simulink model "P_vertical"  (R2017b)
settings: Solver=VariableStepAuto  StartTime=0.0  StopTime=10.0  RelTol=1e-3
libraries: simulink x1
settings Model: Creator=Rita Monteiro  LastModifiedBy=Rita Monteiro

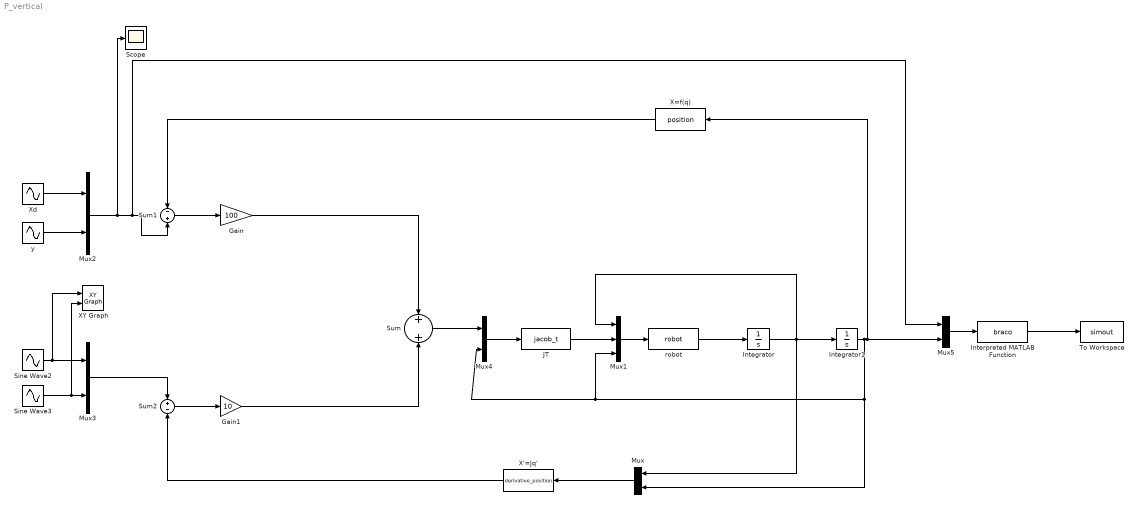
== system P_vertical ==
  Gain : Gain  Gain=100
  Gain1 : Gain  Gain=10
  Integrator : Integrator  InitialCondition=[0;0]
  Integrator1 : Integrator  InitialCondition=[pi/2;-pi/4]
  Interpreted MATLAB Function : MATLABFcn  MATLABFcn=braco  OutputDimensions=1
  JT : MATLABFcn  MATLABFcn=jacob_t  OutputDimensions=2
  Mux{,2..5} (5 alike) : Mux  Inputs=2
  Mux1 : Mux  Inputs=3
  Scope : Scope
  Sine Wave2 : Sin  Amplitude=0  Frequency=2*pi*0.25  Phase=pi  SampleTime=0
  Sine Wave3 : Sin  Amplitude=0.07*(2*pi*0.25)  Frequency=2*pi*0.25  Phase=pi/2  SampleTime=0
  Sum : Sum
  Sum1 : Sum  Inputs=-|+
  Sum2 : Sum  Inputs=+|-
  To Workspace : ToWorkspace  VariableName=simout  SampleTime=-1
  X'=Jq' : MATLABFcn  MATLABFcn=derivative_position
  X=f(q) : MATLABFcn  MATLABFcn=position
  XY Graph : simulink/Sinks/XY Graph  xmin=-1  xmax=1  ymin=-1  ymax=1  st=-1
  Xd : Sin  Amplitude=0  Bias=0.25  Frequency=2*pi*0.25  Phase=pi/2  SampleTime=0
  robot : MATLABFcn  MATLABFcn=robot  OutputDimensions=2
  y : Sin  Amplitude=0.07  Bias=0.2  Frequency=2*pi*(1/4)  SampleTime=0
  wires:
  X'=Jq'/1 -> Sum2/2
  X=f(q)/1 -> Sum1/1
  Sum/1 -> Mux4/1
  Mux4/1 -> JT/1
  Mux1/1 -> robot/1
  Mux5/1 -> Interpreted MATLAB Function/1
  JT/1 -> Mux1/2
  Sum1/1 -> Gain/1
  Interpreted MATLAB Function/1 -> To Workspace/1
  Mux3/1 -> Sum2/1
  Mux2/1 -> Sum1/2, Mux5/1, Scope/1
  Gain1/1 -> Sum/2
  Mux/1 -> X'=Jq'/1
  robot/1 -> Integrator/1
  Integrator1/1 -> Mux5/2, X=f(q)/1, Mux4/2, Mux1/3, Mux/2
  Integrator/1 -> Mux/1, Mux1/1, Integrator1/1
  Sine Wave3/1 -> XY Graph/2, Mux3/2
  Xd/1 -> Mux2/1
  Sum2/1 -> Gain1/1
  Gain/1 -> Sum/1
  Sine Wave2/1 -> XY Graph/1, Mux3/1
  y/1 -> Mux2/2
